simulink model "TC_organized"  (R2026a)
settings: Solver=FixedStepDiscrete  StopTime=timeMax  FixedStep=Ts_plant
InitFcn:
  | TC_paramsOnly = true;
  | run('params.m');
  | clear TC_paramsOnly
values from neighbouring files (symbols this model uses):
  aeroFrontFraction = 0.50    (= 0.5)    [TC_parameters.m]    (also in params.m; params_track.m)
  CDA = 1.20    (= 1.2)    [TC_parameters.m]    (also in params.m; params_track.m)
  CLA = 4.40    (= 4.4)    [TC_parameters.m]    (also in params.m; params_track.m)
  Cmax = 0    [TC_parameters.m]    (also in params.m = 5.375; params_track.m = 5.375)
  Cmin = -Max_Motor_Torque    (= -21.5)    [TC_parameters.m]    (also in params.m; params_track.m)
  distanceTarget = 75    [TC_parameters.m]    (also in params.m)
  Drive_Train = 0.85    [TC_parameters.m]    (also in params.m = 0.92; params_track.m = 0.92)
  fd = 12.5    [TC_parameters.m]    (also in params.m; params_track.m)
  Feedforward_FallRate_FL = 2000    [params.m]    (also in params_track.m)
  Feedforward_FallRate_FR = 2000    [params.m]    (also in params_track.m)
  Feedforward_FallRate_RL = 2000    [params.m]    (also in params_track.m)
  Feedforward_FallRate_RR = 2000    [params.m]    (also in params_track.m)
  Feedforward_Filter_Alpha = 1 - exp(-2*pi*Feedforward_Filter_Hz*Ts)    [params.m]    (also in params_track.m)
  Feedforward_InitialState_FL = muFz_front_launch / Feedforward_Filter_Alpha    [params.m]    (also in params_track.m)
  Feedforward_InitialState_FR = Feedforward_InitialState_FL    [params.m]    (also in params_track.m)
  Feedforward_InitialState_RL = muFz_rear_launch / Feedforward_Filter_Alpha    [params.m]    (also in params_track.m)
  Feedforward_InitialState_RR = Feedforward_InitialState_RL    [params.m]    (also in params_track.m)
  Feedforward_Launch_FL = min(Max_Motor_Torque, Kff_FL*r/(fd*Drive_Train) *      muFz_front_launch*targetForceShape(Slip_Target_FL))    [params.m]    (also in params_track.m)
  Feedforward_Launch_FR = min(Max_Motor_Torque, Kff_FR*r/(fd*Drive_Train) *      muFz_front_launch*targetForceShape(Slip_Target_FR))    [params.m]    (also in params_track.m)
  Feedforward_Launch_RL = min(Max_Motor_Torque, Kff_RL*r/(fd*Drive_Train) *      muFz_rear_launch*targetForceShape(Slip_Target_RL))    [params.m]    (also in params_track.m)
  Feedforward_Launch_RR = min(Max_Motor_Torque, Kff_RR*r/(fd*Drive_Train) *      muFz_rear_launch*targetForceShape(Slip_Target_RR))    [params.m]    (also in params_track.m)
  Feedforward_RiseRate_FL = 800    [params.m]    (also in params_track.m)
  Feedforward_RiseRate_FR = 800    [params.m]    (also in params_track.m)
  Feedforward_RiseRate_RL = 800    [params.m]    (also in params_track.m)
  Feedforward_RiseRate_RR = 800    [params.m]    (also in params_track.m)
  Fz_front_static = Mv * gravity * cg_r / W    (= 1387.6672151)    [TC_parameters.m]    (also in params.m; params_track.m)
  Fz_rear_static = Mv * gravity * cg_f / W    (= 1387.6672151)    [TC_parameters.m]    (also in params.m; params_track.m)
  Grip_Fact = 1.0    (= 1)    [TC_parameters.m]    (also in params.m = 0.6; params_track.m = 0.6)
  h_cg = 10.4 * in_to_m    (= 0.26416)    [TC_parameters.m]    (also in params.m; params_track.m)
  J_wheel_side = 0.45    [TC_parameters.m]    (also in params.m = 0.35; params_track.m = 0.35)
  Kaw_FL = Ki_FL / Kp_FL    (= 32)    [params.m]    (also in params_track.m)
  Kaw_FR = Ki_FR / Kp_FR    (= 32)    [params.m]    (also in params_track.m)
  Kaw_RL = Ki_RL / Kp_RL    (= 12)    [params.m]    (also in params_track.m)
  Kaw_RR = Ki_RR / Kp_RR    (= 12)    [params.m]    (also in params_track.m)
  Kd_FL = 0    [TC_parameters.m]    (also in params.m; params_track.m)
  Kd_FR = 0    [TC_parameters.m]    (also in params.m; params_track.m)
  Kd_RL = 0    [TC_parameters.m]    (also in params.m; params_track.m)
  Kd_RR = 0    [TC_parameters.m]    (also in params.m; params_track.m)
  Kff_FL = 0.9    [params.m]    (also in params_track.m)
  Kff_FR = 0.9    [params.m]    (also in params_track.m)
  Kff_RL = 0.9    [params.m]    (also in params_track.m)
  Kff_RR = 0.9    [params.m]    (also in params_track.m)
  Ki_FL = 180    [TC_parameters.m]    (also in params.m = 480; params_track.m = 480)
  Ki_FR = 180    [TC_parameters.m]    (also in params.m = 480; params_track.m = 480)
  Ki_RL = 180    [TC_parameters.m]    (also in params.m = 240; params_track.m = 240)
  Ki_RR = 180    [TC_parameters.m]    (also in params.m = 240; params_track.m = 240)
  Kp_FL = 32    [TC_parameters.m]    (also in params.m = 15; params_track.m = 15)
  Kp_FR = 32    [TC_parameters.m]    (also in params.m = 15; params_track.m = 15)
  Kp_RL = 32    [TC_parameters.m]    (also in params.m = 20; params_track.m = 20)
  Kp_RR = 32    [TC_parameters.m]    (also in params.m = 20; params_track.m = 20)
  Ktrack_FL = 50    [params.m]    (also in params_track.m)
  Ktrack_FR = 50    [params.m]    (also in params_track.m)
  Ktrack_RL = 50    [params.m]    (also in params_track.m)
  Ktrack_RR = 50    [params.m]    (also in params_track.m)
  Launch_Pedal_Initial = T_request_per_motor    (= 21.5)    [params.m]    (also in params_track.m)
  Max_Motor_Torque = 21.5    [TC_parameters.m]    (also in params.m; params_track.m)
  Max_Wheel_Omega = Max_Motor_RPM * 2*pi/60 / fd    (= 167.551608191)    [TC_parameters.m]    (also in params.m; params_track.m)
  maxTractivePower = 80e3    (= 80000)    [TC_parameters.m]    (also in params.m; params_track.m)
  motorInverterEfficiency = 1.00    (= 1)    [params.m]    (also in params_track.m)
  Mv = vehicleMassNoDriver + driverMass    (= 283.00535149)    [TC_parameters.m]    (also in params.m; params_track.m)
  Pacejka_B = 10.400    (= 10.4)    [TC_parameters.m]    (also in params.m; params_track.m)
  Pacejka_C = -1.580    (= -1.58)    [TC_parameters.m]    (also in params.m; params_track.m)
  Pacejka_D1 = -3.020    (= -3.02)    [TC_parameters.m]    (also in params.m; params_track.m)
  Pacejka_D2 = 0.800    (= 0.8)    [TC_parameters.m]    (also in params.m; params_track.m)
  r = 0.5 * 16.0 * in_to_m    (= 0.2032)    [TC_parameters.m]    (also in params.m; params_track.m; slip_estimator.m = ay / vref0)
  rho = 1.225    [TC_parameters.m]    (also in params.m; params_track.m)
  Slip_Filter_Alpha = 1 - exp(-2*pi*Slip_Filter_Hz*Ts)    [params.m]    (also in params_track.m)
  Slip_Target_FL = 0.12    [TC_parameters.m]    (also in params.m; params_track.m)
  Slip_Target_FR = 0.12    [TC_parameters.m]    (also in params.m; params_track.m)
  Slip_Target_RL = 0.12    [TC_parameters.m]    (also in params.m = 0.145; params_track.m = 0.145)
  Slip_Target_RR = 0.12    [TC_parameters.m]    (also in params.m = 0.145; params_track.m = 0.145)
  slipSpeedFloor = 0.50    (= 0.5)    [TC_parameters.m]    (also in params.m; params_track.m)
  Speed_Limit_Taper_Omega = Speed_Limit_Taper_RPM * 2*pi/60 / fd    (= 4.18879020479)    [params.m]    (also in params_track.m)
  T_request_per_motor = Max_Motor_Torque    (= 21.5)    [TC_parameters.m]    (also in params.m; params_track.m)
  tau_motor = 0.03    [TC_parameters.m]    (also in params.m = 0.005; params_track.m = 0.005)
  Ts = 0.002    [TC_parameters.m]    (also in params.m; params_track.m)
  Ts_plant = 0.0001    [params.m]    (also in params_track.m)
  W = 60.25 * in_to_m    (= 1.53035)    [TC_parameters.m]    (also in params.m; params_track.m)
undefined symbols (not defined in the file or in its folder): DiscIntNeverNeededParam
libraries: slpidlib x4
(part 2 of 2)

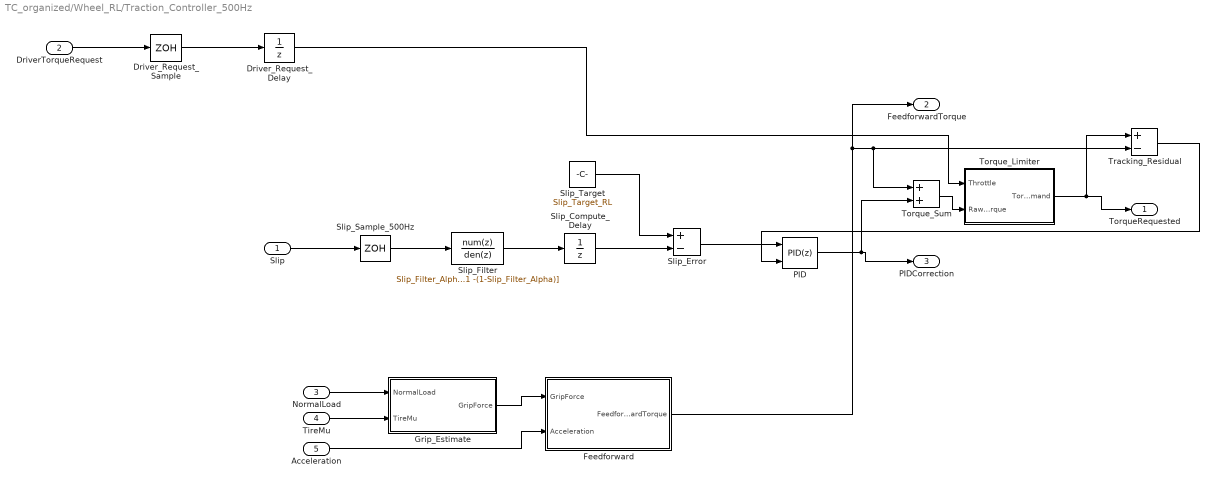
== system TC_organized/Wheel_RL/Traction_Controller_500Hz ==
  Slip : Inport
  DriverTorqueRequest : Inport  Port=2
  NormalLoad : Inport  Port=3
  TireMu : Inport  Port=4
  Acceleration : Inport  Port=5
  Driver_Request_Delay : UnitDelay  InitialCondition=Launch_Pedal_Initial  SampleTime=Ts
  Driver_Request_Sample : ZeroOrderHold  SampleTime=Ts
  Feedforward : Subsystem
  Grip_Estimate : Subsystem
  PID : slpidlib/PID Controller  Controller=PID  Form=Parallel  TimeDomain=Discrete-time  UseExternalTs=off  SampleTime=Ts  IntegratorMethod=Forward Euler  FilterMethod=Forward Euler  ControllerParametersSource=internal  P=Kp_RL  I=Ki_RL  UseKiTs=off  D=Kd_RL  UseExternalDerivativeSource=off  N=100  UseFilter=on  TunerSelectOption=Transfer Function Based (PID Tuner App)  InitialConditionSource=internal  InitialConditionForIntegrator=0  InitialConditionForFilter=0  DifferentiatorICPrevScaledInput=0  ExternalReset=none  TrackingMode=on  Kt=Ktrack_RL  LimitOutput=on  SatLimitsSource=internal  UpperSaturationLimit=Cmax  LowerSaturationLimit=Cmin  LinearizeAsGain=on  AntiWindupMode=back-calculation  Kb=Kaw_RL  LimitIntegrator=off  UpperIntegratorSaturationLimit=inf  LowerIntegratorSaturationLimit=-inf  POutMin=[]  POutMax=[]  IOutMin=[]  IOutMax=[]  DOutMin=[]  DOutMax=[]  NOutMin=[]  NOutMax=[]  SumOutMin=[]  SumOutMax=[]  SaturationOutMin=[]  SaturationOutMax=[]  PParamMin=[]  PParamMax=[]  IParamMin=[]  IParamMax=[]  DParamMin=[]  DParamMax=[]  NParamMin=[]  NParamMax=[]  KbParamMin=[]  KbParamMax=[]  KtParamMin=[]  KtParamMax=[]  KbOutMin=[]  KbOutMax=[]  KtOutMin=[]  KtOutMax=[]  IntegratorOutMin=[]  IntegratorOutMax=[]  FilterOutMin=[]  FilterOutMax=[]  SumI1OutMin=[]  SumI1OutMax=[]  SumI2OutMin=[]  SumI2OutMax=[]  SumI3OutMin=[]  SumI3OutMax=[]  SumI4OutMin=[]  SumI4OutMax=[]  SumDOutMin=[]  SumDOutMax=[]  DifferentiatorOutMin=[]  DifferentiatorOutMax=[]  FilterDiffOutCoefMin=[]  FilterDiffOutCoefMax=[]  ReciprocalOutMin=[]  ReciprocalOutMax=[]  SumDenOutMin=[]  SumDenOutMax=[]  SumNumOutMin=[]  SumNumOutMax=[]  DivideOutMin=[]  DivideOutMax=[]  UdiffTsProdOutMin=[]  UdiffTsProdOutMax=[]  NTsProdOutMin=[]  NTsProdOutMax=[]  UintegralTsProdOutMin=[]  UintegralTsProdOutMax=[]  UngainTsProdOutMin=[]  UngainTsProdOutMax=[]  ClampingZeroOutDataTypeStr=Inherit: Inherit via back propagation  ClampingZeroOutMin=[]  ClampingZeroOutMax=[]  FilterDenConstantOutDataTypeStr=Inherit: Inherit via back propagation  FilterDenConstantOutMin=[]  FilterDenConstantOutMax=[]  PCopyOutDataTypeStr=Inherit: Inherit via back propagation  PCopyOutMin=[]  PCopyOutMax=[]  NCopyOutDataTypeStr=Inherit: Inherit via back propagation  NCopyOutMin=[]  NCopyOutMax=[]  IntegratorContinuousStateAttributes=''  IntegratorStateMustResolveToSignalObject=off  IntegratorRTWStateStorageClass=Auto  FilterContinuousStateAttributes=''  FilterStateMustResolveToSignalObject=off  FilterRTWStateStorageClass=Auto  ParallelPVariant=InternalParameters  IdealPVariant=Disabled  IVariant=InternalParameters  DVariant=InternalParameters  IntegratorVariant=Discrete  SatVariant=Enabled  AWVariant=BackCalculation  PCopyVariant=Disabled  TRVariant=Enabled  FdbkBlocksVariant=Forward  IdealPFdbkVariant=Disabled  SatFdbkVariant=Disabled  DerivativeFilterVariant=ForwardEulerFilter  NVariant=InternalParameters  NCopyVariant=Disabled  FilterICVariant=InternalICsFilter  IntegratorICVariant=InternalICs  ExternalResetVariant=Disabled  TRSumVariant=TrackingMode  SumFdbkVariant=Disabled  SumVariant=Sum_PID  TsampFilterVariant=InternalTs  TsampNgainVariant=Passthrough  TsampIntegralVariant=Disabled_SignalSpec  ExternalSaturationOutDataTypeStr=Inherit: Same as second input  DerivativeSourceVariant=ErrorSignal  PreIntVariant=InternalPreInt
  Slip_Compute_Delay : UnitDelay  SampleTime=Ts
  Slip_Error : Sum  Inputs=+-
  Slip_Filter : DiscreteFilter  Numerator=Slip_Filter_Alpha  Denominator=[1 -(1-Slip_Filter_Alpha)]  SampleTime=Ts
  Slip_Sample_500Hz : ZeroOrderHold  SampleTime=Ts
  Slip_Target : Constant  Value=Slip_Target_RL
  Torque_Limiter : Subsystem
  Torque_Sum : Sum
  Tracking_Residual : Sum  Inputs=+-
  TorqueRequested : Outport
  FeedforwardTorque : Outport  Port=2
  PIDCorrection : Outport  Port=3
  wires:
  Tracking_Residual/1 -> PID/2
  PID/1 -> Torque_Sum/2, PIDCorrection/1
  Driver_Request_Sample/1 -> Driver_Request_Delay/1
  DriverTorqueRequest/1 -> Driver_Request_Sample/1
  Slip_Error/1 -> PID/1
  Slip_Compute_Delay/1 -> Slip_Error/2
  Slip_Target/1 -> Slip_Error/1
  Slip_Filter/1 -> Slip_Compute_Delay/1
  Slip_Sample_500Hz/1 -> Slip_Filter/1
  Slip/1 -> Slip_Sample_500Hz/1
  Feedforward/1(FeedforwardTorque) -> Torque_Sum/1, Tracking_Residual/2, FeedforwardTorque/1
  NormalLoad/1 -> Grip_Estimate/1(NormalLoad)
  TireMu/1 -> Grip_Estimate/2(TireMu)
  Grip_Estimate/1(GripForce) -> Feedforward/1(GripForce)
  Acceleration/1 -> Feedforward/2(Acceleration)
  Torque_Limiter/1(TorqueCommand) -> Tracking_Residual/1, TorqueRequested/1
  Driver_Request_Delay/1 -> Torque_Limiter/1(Throttle)
  Torque_Sum/1 -> Torque_Limiter/2(RawTorque)

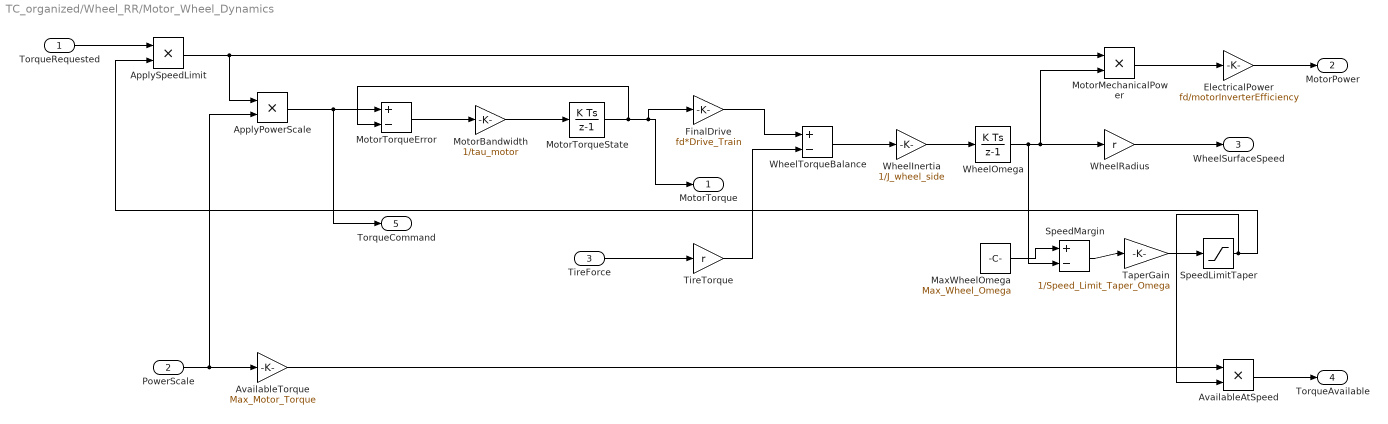
== system TC_organized/Wheel_RR/Motor_Wheel_Dynamics ==
  TorqueRequested : Inport
  PowerScale : Inport  Port=2
  TireForce : Inport  Port=3
  ApplyPowerScale : Product  Inputs=**
  ApplySpeedLimit : Product  Inputs=**
  AvailableAtSpeed : Product  Inputs=**
  AvailableTorque : Gain  Gain=Max_Motor_Torque
  ElectricalPower : Gain  Gain=fd/motorInverterEfficiency
  FinalDrive : Gain  Gain=fd*Drive_Train
  MaxWheelOmega : Constant  Value=Max_Wheel_Omega
  MotorBandwidth : Gain  Gain=1/tau_motor
  MotorMechanicalPower : Product  Inputs=**
  MotorTorqueError : Sum  Inputs=+-
  MotorTorqueState : DiscreteIntegrator  SampleTime=Ts_plant  ICPrevOutput=DiscIntNeverNeededParam  ICPrevScaledInput=DiscIntNeverNeededParam
  SpeedLimitTaper : Saturate  UpperLimit=1  LowerLimit=0
  SpeedMargin : Sum  Inputs=+-
  TaperGain : Gain  Gain=1/Speed_Limit_Taper_Omega
  TireTorque : Gain  Gain=r
  WheelInertia : Gain  Gain=1/J_wheel_side
  WheelOmega : DiscreteIntegrator  SampleTime=Ts_plant  ICPrevOutput=DiscIntNeverNeededParam  ICPrevScaledInput=DiscIntNeverNeededParam
  WheelRadius : Gain  Gain=r
  WheelTorqueBalance : Sum  Inputs=+-
  MotorTorque : Outport
  MotorPower : Outport  Port=2
  WheelSurfaceSpeed : Outport  Port=3
  TorqueAvailable : Outport  Port=4
  TorqueCommand : Outport  Port=5
  wires:
  AvailableAtSpeed/1 -> TorqueAvailable/1
  WheelRadius/1 -> WheelSurfaceSpeed/1
  ElectricalPower/1 -> MotorPower/1
  MotorMechanicalPower/1 -> ElectricalPower/1
  WheelInertia/1 -> WheelOmega/1
  WheelTorqueBalance/1 -> WheelInertia/1
  TireTorque/1 -> WheelTorqueBalance/2
  FinalDrive/1 -> WheelTorqueBalance/1
  TireForce/1 -> TireTorque/1
  MotorBandwidth/1 -> MotorTorqueState/1
  MotorTorqueError/1 -> MotorBandwidth/1
  MotorTorqueState/1 -> FinalDrive/1, MotorTorque/1, MotorTorqueError/2
  ApplyPowerScale/1 -> MotorTorqueError/1, TorqueCommand/1
  ApplySpeedLimit/1 -> ApplyPowerScale/1, MotorMechanicalPower/1
  AvailableTorque/1 -> AvailableAtSpeed/1
  PowerScale/1 -> ApplyPowerScale/2, AvailableTorque/1
  WheelOmega/1 -> MotorMechanicalPower/2, WheelRadius/1, SpeedMargin/2
  TorqueRequested/1 -> ApplySpeedLimit/1
  MaxWheelOmega/1 -> SpeedMargin/1
  SpeedMargin/1 -> TaperGain/1
  TaperGain/1 -> SpeedLimitTaper/1
  SpeedLimitTaper/1 -> ApplySpeedLimit/2, AvailableAtSpeed/2

== system TC_organized/Wheel_RR/Slip_Estimator ==
  VehicleSpeed : Inport
  WheelSurfaceSpeed : Inport  Port=2
  SlipDenominator : MinMax  Function=max  Inputs=2
  SlipNumerator : Sum  Inputs=+-
  SlipRatio : Product  Inputs=*/
  SlipSpeedFloor : Constant  Value=slipSpeedFloor
  Slip : Outport
  wires:
  SlipRatio/1 -> Slip/1
  SlipDenominator/1 -> SlipRatio/2
  SlipNumerator/1 -> SlipRatio/1
  SlipSpeedFloor/1 -> SlipDenominator/2
  VehicleSpeed/1 -> SlipDenominator/1, SlipNumerator/2
  WheelSurfaceSpeed/1 -> SlipNumerator/1

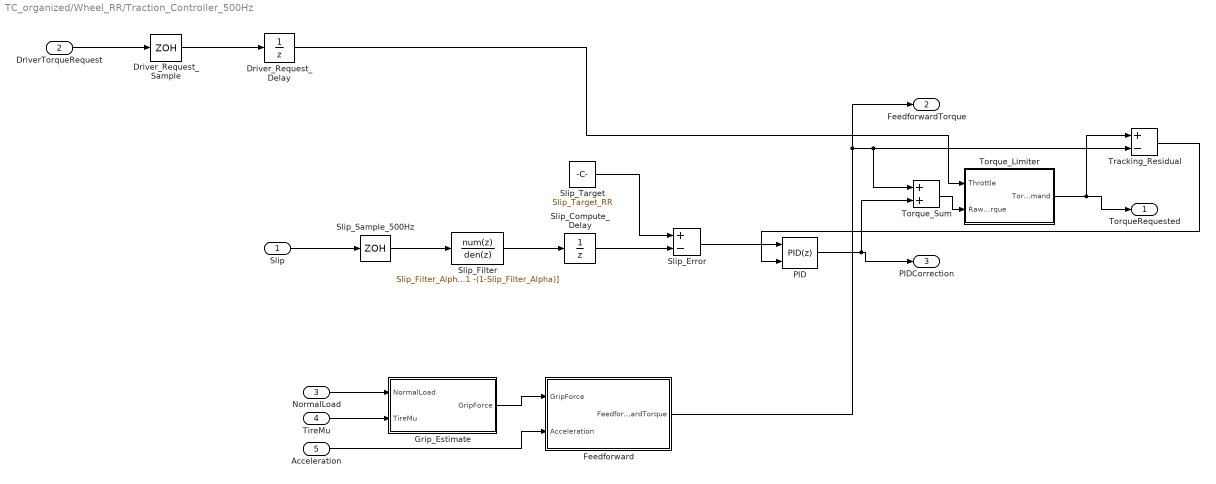
== system TC_organized/Wheel_RR/Traction_Controller_500Hz ==
  Slip : Inport
  DriverTorqueRequest : Inport  Port=2
  NormalLoad : Inport  Port=3
  TireMu : Inport  Port=4
  Acceleration : Inport  Port=5
  Driver_Request_Delay : UnitDelay  InitialCondition=Launch_Pedal_Initial  SampleTime=Ts
  Driver_Request_Sample : ZeroOrderHold  SampleTime=Ts
  Feedforward : Subsystem
  Grip_Estimate : Subsystem
  PID : slpidlib/PID Controller  Controller=PID  Form=Parallel  TimeDomain=Discrete-time  UseExternalTs=off  SampleTime=Ts  IntegratorMethod=Forward Euler  FilterMethod=Forward Euler  ControllerParametersSource=internal  P=Kp_RR  I=Ki_RR  UseKiTs=off  D=Kd_RR  UseExternalDerivativeSource=off  N=100  UseFilter=on  TunerSelectOption=Transfer Function Based (PID Tuner App)  InitialConditionSource=internal  InitialConditionForIntegrator=0  InitialConditionForFilter=0  DifferentiatorICPrevScaledInput=0  ExternalReset=none  TrackingMode=on  Kt=Ktrack_RR  LimitOutput=on  SatLimitsSource=internal  UpperSaturationLimit=Cmax  LowerSaturationLimit=Cmin  LinearizeAsGain=on  AntiWindupMode=back-calculation  Kb=Kaw_RR  LimitIntegrator=off  UpperIntegratorSaturationLimit=inf  LowerIntegratorSaturationLimit=-inf  POutMin=[]  POutMax=[]  IOutMin=[]  IOutMax=[]  DOutMin=[]  DOutMax=[]  NOutMin=[]  NOutMax=[]  SumOutMin=[]  SumOutMax=[]  SaturationOutMin=[]  SaturationOutMax=[]  PParamMin=[]  PParamMax=[]  IParamMin=[]  IParamMax=[]  DParamMin=[]  DParamMax=[]  NParamMin=[]  NParamMax=[]  KbParamMin=[]  KbParamMax=[]  KtParamMin=[]  KtParamMax=[]  KbOutMin=[]  KbOutMax=[]  KtOutMin=[]  KtOutMax=[]  IntegratorOutMin=[]  IntegratorOutMax=[]  FilterOutMin=[]  FilterOutMax=[]  SumI1OutMin=[]  SumI1OutMax=[]  SumI2OutMin=[]  SumI2OutMax=[]  SumI3OutMin=[]  SumI3OutMax=[]  SumI4OutMin=[]  SumI4OutMax=[]  SumDOutMin=[]  SumDOutMax=[]  DifferentiatorOutMin=[]  DifferentiatorOutMax=[]  FilterDiffOutCoefMin=[]  FilterDiffOutCoefMax=[]  ReciprocalOutMin=[]  ReciprocalOutMax=[]  SumDenOutMin=[]  SumDenOutMax=[]  SumNumOutMin=[]  SumNumOutMax=[]  DivideOutMin=[]  DivideOutMax=[]  UdiffTsProdOutMin=[]  UdiffTsProdOutMax=[]  NTsProdOutMin=[]  NTsProdOutMax=[]  UintegralTsProdOutMin=[]  UintegralTsProdOutMax=[]  UngainTsProdOutMin=[]  UngainTsProdOutMax=[]  ClampingZeroOutDataTypeStr=Inherit: Inherit via back propagation  ClampingZeroOutMin=[]  ClampingZeroOutMax=[]  FilterDenConstantOutDataTypeStr=Inherit: Inherit via back propagation  FilterDenConstantOutMin=[]  FilterDenConstantOutMax=[]  PCopyOutDataTypeStr=Inherit: Inherit via back propagation  PCopyOutMin=[]  PCopyOutMax=[]  NCopyOutDataTypeStr=Inherit: Inherit via back propagation  NCopyOutMin=[]  NCopyOutMax=[]  IntegratorContinuousStateAttributes=''  IntegratorStateMustResolveToSignalObject=off  IntegratorRTWStateStorageClass=Auto  FilterContinuousStateAttributes=''  FilterStateMustResolveToSignalObject=off  FilterRTWStateStorageClass=Auto  ParallelPVariant=InternalParameters  IdealPVariant=Disabled  IVariant=InternalParameters  DVariant=InternalParameters  IntegratorVariant=Discrete  SatVariant=Enabled  AWVariant=BackCalculation  PCopyVariant=Disabled  TRVariant=Enabled  FdbkBlocksVariant=Forward  IdealPFdbkVariant=Disabled  SatFdbkVariant=Disabled  DerivativeFilterVariant=ForwardEulerFilter  NVariant=InternalParameters  NCopyVariant=Disabled  FilterICVariant=InternalICsFilter  IntegratorICVariant=InternalICs  ExternalResetVariant=Disabled  TRSumVariant=TrackingMode  SumFdbkVariant=Disabled  SumVariant=Sum_PID  TsampFilterVariant=InternalTs  TsampNgainVariant=Passthrough  TsampIntegralVariant=Disabled_SignalSpec  ExternalSaturationOutDataTypeStr=Inherit: Same as second input  DerivativeSourceVariant=ErrorSignal  PreIntVariant=InternalPreInt
  Slip_Compute_Delay : UnitDelay  SampleTime=Ts
  Slip_Error : Sum  Inputs=+-
  Slip_Filter : DiscreteFilter  Numerator=Slip_Filter_Alpha  Denominator=[1 -(1-Slip_Filter_Alpha)]  SampleTime=Ts
  Slip_Sample_500Hz : ZeroOrderHold  SampleTime=Ts
  Slip_Target : Constant  Value=Slip_Target_RR
  Torque_Limiter : Subsystem
  Torque_Sum : Sum
  Tracking_Residual : Sum  Inputs=+-
  TorqueRequested : Outport
  FeedforwardTorque : Outport  Port=2
  PIDCorrection : Outport  Port=3
  wires:
  Tracking_Residual/1 -> PID/2
  PID/1 -> Torque_Sum/2, PIDCorrection/1
  Driver_Request_Sample/1 -> Driver_Request_Delay/1
  DriverTorqueRequest/1 -> Driver_Request_Sample/1
  Slip_Error/1 -> PID/1
  Slip_Compute_Delay/1 -> Slip_Error/2
  Slip_Target/1 -> Slip_Error/1
  Slip_Filter/1 -> Slip_Compute_Delay/1
  Slip_Sample_500Hz/1 -> Slip_Filter/1
  Slip/1 -> Slip_Sample_500Hz/1
  Feedforward/1(FeedforwardTorque) -> Torque_Sum/1, Tracking_Residual/2, FeedforwardTorque/1
  NormalLoad/1 -> Grip_Estimate/1(NormalLoad)
  TireMu/1 -> Grip_Estimate/2(TireMu)
  Grip_Estimate/1(GripForce) -> Feedforward/1(GripForce)
  Acceleration/1 -> Feedforward/2(Acceleration)
  Torque_Limiter/1(TorqueCommand) -> Tracking_Residual/1, TorqueRequested/1
  Driver_Request_Delay/1 -> Torque_Limiter/1(Throttle)
  Torque_Sum/1 -> Torque_Limiter/2(RawTorque)

== system TC_organized/Wheel_FL/Traction_Controller_500Hz/Feedforward ==
  GripForce : Inport
  Acceleration : Inport  Port=2
  Accel_Filter : DiscreteFilter  Numerator=Feedforward_Filter_Alpha  Denominator=[1 -(1-Feedforward_Filter_Alpha)]  SampleTime=Ts
  Accel_Sample_500Hz : ZeroOrderHold  SampleTime=Ts
  Feedforward_Delta : Sum  Inputs=+-
  Feedforward_Limit : Saturate  UpperLimit=Max_Motor_Torque  LowerLimit=0
  Feedforward_Memory : UnitDelay  InitialCondition=Feedforward_Launch_FL  SampleTime=Ts
  Feedforward_Rate_Limit : Saturate  UpperLimit=Feedforward_RiseRate_FL*Ts  LowerLimit=-Feedforward_FallRate_FL*Ts
  Feedforward_Update : Sum
  Force_At_Target_Slip : Gain  Gain=-sin(Pacejka_C*atan(Pacejka_B*Slip_Target_FL))
  Grip_Feedforward : Sum
  Tire_To_Motor_Torque : Gain  Gain=Kff_FL*r/(fd*Drive_Train)
  Wheel_Inertia_FF : Gain  Gain=J_wheel_side/(r*fd*Drive_Train)
  FeedforwardTorque : Outport
  wires:
  GripForce/1 -> Force_At_Target_Slip/1
  Force_At_Target_Slip/1 -> Tire_To_Motor_Torque/1
  Tire_To_Motor_Torque/1 -> Grip_Feedforward/1
  Acceleration/1 -> Accel_Sample_500Hz/1
  Accel_Sample_500Hz/1 -> Accel_Filter/1
  Accel_Filter/1 -> Wheel_Inertia_FF/1
  Wheel_Inertia_FF/1 -> Grip_Feedforward/2
  Grip_Feedforward/1 -> Feedforward_Delta/1
  Feedforward_Memory/1 -> Feedforward_Delta/2, Feedforward_Update/1
  Feedforward_Delta/1 -> Feedforward_Rate_Limit/1
  Feedforward_Rate_Limit/1 -> Feedforward_Update/2
  Feedforward_Update/1 -> Feedforward_Limit/1, Feedforward_Memory/1
  Feedforward_Limit/1 -> FeedforwardTorque/1

== system TC_organized/Wheel_FL/Traction_Controller_500Hz/Grip_Estimate ==
  NormalLoad : Inport
  TireMu : Inport  Port=2
  Grip_Filter : DiscreteFilter  Numerator=Feedforward_Filter_Alpha  Denominator=[1 -(1-Feedforward_Filter_Alpha)]  InitialStates=Feedforward_InitialState_FL  SampleTime=Ts
  Grip_Sample_500Hz : ZeroOrderHold  SampleTime=Ts
  Mu_Times_Load : Product  Inputs=**
  GripForce : Outport
  wires:
  NormalLoad/1 -> Mu_Times_Load/1
  TireMu/1 -> Mu_Times_Load/2
  Mu_Times_Load/1 -> Grip_Sample_500Hz/1
  Grip_Sample_500Hz/1 -> Grip_Filter/1
  Grip_Filter/1 -> GripForce/1

== system TC_organized/Wheel_FL/Traction_Controller_500Hz/Torque_Limiter ==
  Throttle : Inport
  RawTorque : Inport  Port=2
  Pedal_Limit : MinMax  Inputs=2
  Torque_Limit : Saturate  UpperLimit=Max_Motor_Torque  LowerLimit=0
  TorqueCommand : Outport
  wires:
  Torque_Limit/1 -> TorqueCommand/1
  Pedal_Limit/1 -> Torque_Limit/1
  Throttle/1 -> Pedal_Limit/2
  RawTorque/1 -> Pedal_Limit/1

== system TC_organized/Wheel_FR/Traction_Controller_500Hz/Feedforward ==
  GripForce : Inport
  Acceleration : Inport  Port=2
  Accel_Filter : DiscreteFilter  Numerator=Feedforward_Filter_Alpha  Denominator=[1 -(1-Feedforward_Filter_Alpha)]  SampleTime=Ts
  Accel_Sample_500Hz : ZeroOrderHold  SampleTime=Ts
  Feedforward_Delta : Sum  Inputs=+-
  Feedforward_Limit : Saturate  UpperLimit=Max_Motor_Torque  LowerLimit=0
  Feedforward_Memory : UnitDelay  InitialCondition=Feedforward_Launch_FR  SampleTime=Ts
  Feedforward_Rate_Limit : Saturate  UpperLimit=Feedforward_RiseRate_FR*Ts  LowerLimit=-Feedforward_FallRate_FR*Ts
  Feedforward_Update : Sum
  Force_At_Target_Slip : Gain  Gain=-sin(Pacejka_C*atan(Pacejka_B*Slip_Target_FR))
  Grip_Feedforward : Sum
  Tire_To_Motor_Torque : Gain  Gain=Kff_FR*r/(fd*Drive_Train)
  Wheel_Inertia_FF : Gain  Gain=J_wheel_side/(r*fd*Drive_Train)
  FeedforwardTorque : Outport
  wires:
  GripForce/1 -> Force_At_Target_Slip/1
  Force_At_Target_Slip/1 -> Tire_To_Motor_Torque/1
  Tire_To_Motor_Torque/1 -> Grip_Feedforward/1
  Acceleration/1 -> Accel_Sample_500Hz/1
  Accel_Sample_500Hz/1 -> Accel_Filter/1
  Accel_Filter/1 -> Wheel_Inertia_FF/1
  Wheel_Inertia_FF/1 -> Grip_Feedforward/2
  Grip_Feedforward/1 -> Feedforward_Delta/1
  Feedforward_Memory/1 -> Feedforward_Delta/2, Feedforward_Update/1
  Feedforward_Delta/1 -> Feedforward_Rate_Limit/1
  Feedforward_Rate_Limit/1 -> Feedforward_Update/2
  Feedforward_Update/1 -> Feedforward_Limit/1, Feedforward_Memory/1
  Feedforward_Limit/1 -> FeedforwardTorque/1

== system TC_organized/Wheel_FR/Traction_Controller_500Hz/Grip_Estimate ==
  NormalLoad : Inport
  TireMu : Inport  Port=2
  Grip_Filter : DiscreteFilter  Numerator=Feedforward_Filter_Alpha  Denominator=[1 -(1-Feedforward_Filter_Alpha)]  InitialStates=Feedforward_InitialState_FR  SampleTime=Ts
  Grip_Sample_500Hz : ZeroOrderHold  SampleTime=Ts
  Mu_Times_Load : Product  Inputs=**
  GripForce : Outport
  wires:
  NormalLoad/1 -> Mu_Times_Load/1
  TireMu/1 -> Mu_Times_Load/2
  Mu_Times_Load/1 -> Grip_Sample_500Hz/1
  Grip_Sample_500Hz/1 -> Grip_Filter/1
  Grip_Filter/1 -> GripForce/1

== system TC_organized/Wheel_FR/Traction_Controller_500Hz/Torque_Limiter ==
  Throttle : Inport
  RawTorque : Inport  Port=2
  Pedal_Limit : MinMax  Inputs=2
  Torque_Limit : Saturate  UpperLimit=Max_Motor_Torque  LowerLimit=0
  TorqueCommand : Outport
  wires:
  RawTorque/1 -> Pedal_Limit/1
  Throttle/1 -> Pedal_Limit/2
  Pedal_Limit/1 -> Torque_Limit/1
  Torque_Limit/1 -> TorqueCommand/1

== system TC_organized/Wheel_RL/Traction_Controller_500Hz/Feedforward ==
  GripForce : Inport
  Acceleration : Inport  Port=2
  Accel_Filter : DiscreteFilter  Numerator=Feedforward_Filter_Alpha  Denominator=[1 -(1-Feedforward_Filter_Alpha)]  SampleTime=Ts
  Accel_Sample_500Hz : ZeroOrderHold  SampleTime=Ts
  Feedforward_Delta : Sum  Inputs=+-
  Feedforward_Limit : Saturate  UpperLimit=Max_Motor_Torque  LowerLimit=0
  Feedforward_Memory : UnitDelay  InitialCondition=Feedforward_Launch_RL  SampleTime=Ts
  Feedforward_Rate_Limit : Saturate  UpperLimit=Feedforward_RiseRate_RL*Ts  LowerLimit=-Feedforward_FallRate_RL*Ts
  Feedforward_Update : Sum
  Force_At_Target_Slip : Gain  Gain=-sin(Pacejka_C*atan(Pacejka_B*Slip_Target_RL))
  Grip_Feedforward : Sum
  Tire_To_Motor_Torque : Gain  Gain=Kff_RL*r/(fd*Drive_Train)
  Wheel_Inertia_FF : Gain  Gain=J_wheel_side/(r*fd*Drive_Train)
  FeedforwardTorque : Outport
  wires:
  GripForce/1 -> Force_At_Target_Slip/1
  Force_At_Target_Slip/1 -> Tire_To_Motor_Torque/1
  Tire_To_Motor_Torque/1 -> Grip_Feedforward/1
  Acceleration/1 -> Accel_Sample_500Hz/1
  Accel_Sample_500Hz/1 -> Accel_Filter/1
  Accel_Filter/1 -> Wheel_Inertia_FF/1
  Wheel_Inertia_FF/1 -> Grip_Feedforward/2
  Grip_Feedforward/1 -> Feedforward_Delta/1
  Feedforward_Memory/1 -> Feedforward_Delta/2, Feedforward_Update/1
  Feedforward_Delta/1 -> Feedforward_Rate_Limit/1
  Feedforward_Rate_Limit/1 -> Feedforward_Update/2
  Feedforward_Update/1 -> Feedforward_Limit/1, Feedforward_Memory/1
  Feedforward_Limit/1 -> FeedforwardTorque/1

== system TC_organized/Wheel_RL/Traction_Controller_500Hz/Grip_Estimate ==
  NormalLoad : Inport
  TireMu : Inport  Port=2
  Grip_Filter : DiscreteFilter  Numerator=Feedforward_Filter_Alpha  Denominator=[1 -(1-Feedforward_Filter_Alpha)]  InitialStates=Feedforward_InitialState_RL  SampleTime=Ts
  Grip_Sample_500Hz : ZeroOrderHold  SampleTime=Ts
  Mu_Times_Load : Product  Inputs=**
  GripForce : Outport
  wires:
  NormalLoad/1 -> Mu_Times_Load/1
  TireMu/1 -> Mu_Times_Load/2
  Mu_Times_Load/1 -> Grip_Sample_500Hz/1
  Grip_Sample_500Hz/1 -> Grip_Filter/1
  Grip_Filter/1 -> GripForce/1

== system TC_organized/Wheel_RL/Traction_Controller_500Hz/Torque_Limiter ==
  Throttle : Inport
  RawTorque : Inport  Port=2
  Pedal_Limit : MinMax  Inputs=2
  Torque_Limit : Saturate  UpperLimit=Max_Motor_Torque  LowerLimit=0
  TorqueCommand : Outport
  wires:
  Torque_Limit/1 -> TorqueCommand/1
  Pedal_Limit/1 -> Torque_Limit/1
  RawTorque/1 -> Pedal_Limit/1
  Throttle/1 -> Pedal_Limit/2

== system TC_organized/Wheel_RR/Traction_Controller_500Hz/Feedforward ==
  GripForce : Inport
  Acceleration : Inport  Port=2
  Accel_Filter : DiscreteFilter  Numerator=Feedforward_Filter_Alpha  Denominator=[1 -(1-Feedforward_Filter_Alpha)]  SampleTime=Ts
  Accel_Sample_500Hz : ZeroOrderHold  SampleTime=Ts
  Feedforward_Delta : Sum  Inputs=+-
  Feedforward_Limit : Saturate  UpperLimit=Max_Motor_Torque  LowerLimit=0
  Feedforward_Memory : UnitDelay  InitialCondition=Feedforward_Launch_RR  SampleTime=Ts
  Feedforward_Rate_Limit : Saturate  UpperLimit=Feedforward_RiseRate_RR*Ts  LowerLimit=-Feedforward_FallRate_RR*Ts
  Feedforward_Update : Sum
  Force_At_Target_Slip : Gain  Gain=-sin(Pacejka_C*atan(Pacejka_B*Slip_Target_RR))
  Grip_Feedforward : Sum
  Tire_To_Motor_Torque : Gain  Gain=Kff_RR*r/(fd*Drive_Train)
  Wheel_Inertia_FF : Gain  Gain=J_wheel_side/(r*fd*Drive_Train)
  FeedforwardTorque : Outport
  wires:
  GripForce/1 -> Force_At_Target_Slip/1
  Force_At_Target_Slip/1 -> Tire_To_Motor_Torque/1
  Tire_To_Motor_Torque/1 -> Grip_Feedforward/1
  Acceleration/1 -> Accel_Sample_500Hz/1
  Accel_Sample_500Hz/1 -> Accel_Filter/1
  Accel_Filter/1 -> Wheel_Inertia_FF/1
  Wheel_Inertia_FF/1 -> Grip_Feedforward/2
  Grip_Feedforward/1 -> Feedforward_Delta/1
  Feedforward_Memory/1 -> Feedforward_Delta/2, Feedforward_Update/1
  Feedforward_Delta/1 -> Feedforward_Rate_Limit/1
  Feedforward_Rate_Limit/1 -> Feedforward_Update/2
  Feedforward_Update/1 -> Feedforward_Limit/1, Feedforward_Memory/1
  Feedforward_Limit/1 -> FeedforwardTorque/1

== system TC_organized/Wheel_RR/Traction_Controller_500Hz/Grip_Estimate ==
  NormalLoad : Inport
  TireMu : Inport  Port=2
  Grip_Filter : DiscreteFilter  Numerator=Feedforward_Filter_Alpha  Denominator=[1 -(1-Feedforward_Filter_Alpha)]  InitialStates=Feedforward_InitialState_RR  SampleTime=Ts
  Grip_Sample_500Hz : ZeroOrderHold  SampleTime=Ts
  Mu_Times_Load : Product  Inputs=**
  GripForce : Outport
  wires:
  NormalLoad/1 -> Mu_Times_Load/1
  TireMu/1 -> Mu_Times_Load/2
  Mu_Times_Load/1 -> Grip_Sample_500Hz/1
  Grip_Sample_500Hz/1 -> Grip_Filter/1
  Grip_Filter/1 -> GripForce/1

== system TC_organized/Wheel_RR/Traction_Controller_500Hz/Torque_Limiter ==
  Throttle : Inport
  RawTorque : Inport  Port=2
  Pedal_Limit : MinMax  Inputs=2
  Torque_Limit : Saturate  UpperLimit=Max_Motor_Torque  LowerLimit=0
  TorqueCommand : Outport
  wires:
  Pedal_Limit/1 -> Torque_Limit/1
  Torque_Limit/1 -> TorqueCommand/1
  Throttle/1 -> Pedal_Limit/2
  RawTorque/1 -> Pedal_Limit/1

== matlab function TC_organized/Load_Transfer_Predictor/Predict_Loads ==
  data: T_FL input; Fz_FL output; T_FR input; T_RL input; T_RR input; v input; Fz_FR output; Fz_RL output; Fz_RR output; mu_FL output; mu_FR output; mu_RL output; mu_RR output; fd parameter; Drive_Train parameter; r parameter; rho parameter; CDA parameter; CLA parameter; aeroFrontFraction parameter; Mv parameter; J_wheel_side parameter; h_cg parameter; W parameter; Fz_front_static parameter; Fz_rear_static parameter; Pacejka_D1 parameter; Pacejka_D2 parameter; Grip_Fact parameter
function [Fz_FL,Fz_FR,Fz_RL,Fz_RR,mu_FL,mu_FR,mu_RL,mu_RR] = predictLoads(T_FL,T_FR,T_RL,T_RR,v,fd, Drive_Train, r, rho, CDA, CLA, aeroFrontFraction, Mv, J_wheel_side, h_cg, W, Fz_front_static, Fz_rear_static, Pacejka_D1, Pacejka_D2, Grip_Fact)
% Predict normal loads from the commanded motor torques instead of waiting
% for measured acceleration. Wheel inertia adds 4*J/r^2 of equivalent mass.
wheelForce = (T_FL + T_FR + T_RL + T_RR)*fd*Drive_Train/r;
drag = 0.5*rho*CDA*v^2;
aPred = (wheelForce - drag)/(Mv + 4*J_wheel_side/r^2);
transfer = Mv*aPred*h_cg/W;          % Axle load transfer [N]
downforce = 0.5*rho*CLA*v^2;
FzFront = max(0.5*(Fz_front_static + aeroFrontFraction*downforce - transfer), 0);
FzRear = max(0.5*(Fz_rear_static + (1 - aeroFrontFraction)*downforce + transfer), 0);
muFront = max(-(Pacejka_D1 + Pacejka_D2*FzFront/1000)*Grip_Fact, 0);
muRear = max(-(Pacejka_D1 + Pacejka_D2*FzRear/1000)*Grip_Fact, 0);
Fz_FL = FzFront; Fz_FR = FzFront; Fz_RL = FzRear; Fz_RR = FzRear;
mu_FL = muFront; mu_FR = muFront; mu_RL = muRear; mu_RR = muRear;
end

== matlab function TC_organized/Pacejka_Tire_Model ==
  data: slip_FL input; Fx_FL output; slip_FR input; slip_RL input; slip_RR input; Fz_FL input; Fz_FR input; Fz_RL input; Fz_RR input; gripFact input; Fx_FR output; Fx_RL output; Fx_RR output; mu_FL output; mu_FR output; mu_RL output; mu_RR output; Pacejka_B parameter; Pacejka_C parameter; Pacejka_D1 parameter; Pacejka_D2 parameter
function [Fx_FL,Fx_FR,Fx_RL,Fx_RR,mu_FL,mu_FR,mu_RL,mu_RR] = calculatePacejkaFx4(slip_FL,slip_FR,slip_RL,slip_RR,Fz_FL,Fz_FR,Fz_RL,Fz_RR,gripFact,Pacejka_B, Pacejka_C, Pacejka_D1, Pacejka_D2)
% Longitudinal Pacejka tire model. B, C, D1, and D2 are block parameters
% resolved from params.m, so the plant and controller share one tire fit.
slip = [slip_FL slip_FR slip_RL slip_RR];
Fz = max([Fz_FL Fz_FR Fz_RL Fz_RR], 0);
Fz_kN = Fz/1000;
muVec = max(-(Pacejka_D1 + Pacejka_D2.*Fz_kN).*gripFact, 0);
FxVec = -muVec.*Fz.*sin(Pacejka_C.*atan(Pacejka_B.*slip));
Fx_FL = FxVec(1); Fx_FR = FxVec(2);
Fx_RL = FxVec(3); Fx_RR = FxVec(4);
mu_FL = muVec(1); mu_FR = muVec(2);
mu_RL = muVec(3); mu_RR = muVec(4);
end
